simulink model "zoom_adc_single_pol"  (Simulink 7.8)
settings: Solver=FixedStepDiscrete  SolverMode=SingleTasking  StartTime=0.0  StopTime=4096  RelTol=1e-3
undefined symbols (not defined in the file): pfb_coeff_gen_calc
libraries: xbsIndex_r4 x1083, casper_library_misc x66, casper_library_delays x56, xps_library x25, simulink x1
(part 1 of 11)
settings Model: Creator=jayanth  LastModifiedBy=dprice
settings Model: ModifiedComment=|
  | dprice -- Tue Apr 16 12:08:08 2013 -- Version 1.114
  | 
  | First commit at Parkes, 16th April 2013. Just added in the FFT wideband black box, as I've tested this FFT and have faith that it works.
settings Model: ModifiedHistory=|
  | dprice -- Tue Apr 16 12:08:08 2013 -- Version 1.114
  | 
  | First commit at Parkes, 16th April 2013. Just added in the FFT wideband black box, as I've tested this FFT and have faith that it works.
settings DebuggingCC: FcnCallInpInsideContextMsg=Use local settings

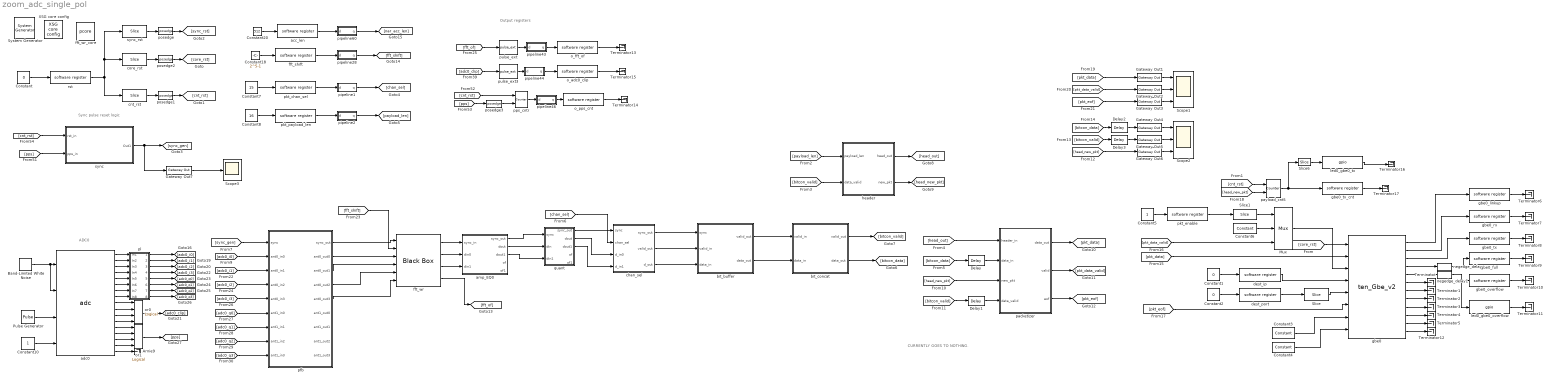
== system zoom_adc_single_pol ==
  note: Sync pulse reset logic
  note: CURRENTLY GOES TO NOTHING.
  note: ADC0
  note: Output registers
  " System Generator" : xbsIndex_r4/ System Generator  Tag=genX  xilinxfamily=virtex5  part=xc5vsx95t  speed=-1  package=ff1136  synthesis_tool=XST  clock_wrapper=Clock Enables  directory=./zoom_adc_single_pol/sysgen  proj_type=Project Navigator  Synth_file=XST Defaults  Impl_file=ISE Defaults  testbench=off  simulink_period=1  sysclk_period=5  dcm_input_clock_period=100  incr_netlist=off  trim_vbits=Everywhere in SubSystem  dbl_ovrd=According to Block Masks  core_generation=According to Block Masks  run_coregen=off  deprecated_control=off  eval_field=0  block_type=sysgen
  Arnie9 : Terminator
  Band-Limited White Noise : simulink/Sources/Band-Limited White Noise  Cov=[0.1]  Ts=0.1  seed=[23341]
  Constant : Constant  Value=0
  Constant1 : Constant  Value=0
  Constant10 : Constant
  Constant18 : Constant  Value=2^5-1
  Constant2 : Constant  Value=0
  Constant20 : Constant  Value=512
  Constant3 : xbsIndex_r4/Constant  const=1  gui_display_data_type=Boolean  arith_type=Boolean  n_bits=16  bin_pt=14  preci_type=Single  exp_width=8  frac_width=24  explicit_period=on  period=1  equ=P=C  opselect=C  inp2=PCIN>>17  opr=+  inp1=P  carry=CIN  dbl_ovrd=off  block_type=constant
  Constant4 : xbsIndex_r4/Constant  const=0  gui_display_data_type=Boolean  arith_type=Boolean  n_bits=16  bin_pt=14  preci_type=Single  exp_width=8  frac_width=24  explicit_period=on  period=1  equ=P=C  opselect=C  inp2=PCIN>>17  opr=+  inp1=P  carry=CIN  dbl_ovrd=off  block_type=constant
  Constant5 : Constant
  Constant6 : xbsIndex_r4/Constant  const=0  gui_display_data_type=Boolean  arith_type=Boolean  n_bits=16  bin_pt=14  preci_type=Single  exp_width=8  frac_width=24  explicit_period=off  period=1  equ=P=C  opselect=C  inp2=PCIN>>17  opr=+  inp1=P  carry=CIN  dbl_ovrd=off  block_type=constant
  Constant7 : Constant  Value=15
  Constant8 : Constant  Value=16
  Delay{,1..3} (4 alike) : xbsIndex_r4/Delay  rst=off  infoeditControl=Selection of Reset will increase slice count due to use of real FFs and instead of SRLs  en=off  latency=1  dbl_ovrd=off  reg_retiming=off  block_type=delay
  Gateway Out{1..7} (7 alike) : xbsIndex_r4/Gateway Out  inherit_from_input=off  hdl_port=on  timing_constraint=None  locs_specified=off  LOCs={}  UseAsDAC=off  DACChannel='1'  block_type=gatewayout
      settings: infoedit="Gateway out block.  Converts Xilinx fixed-point or floating-point type inputs into ouputs of type Simulink integer, single, double, or fixed point.<br><br>Hardware notes:  In hardware these blocks become top level output ports or are discarded, depending on how they are configured."
  Mux : xbsIndex_r4/Mux  inputs=2  en=off  latency=0  precision=Full  arith_type=Unsigned  n_bits=16  bin_pt=14  quantization=Truncate  overflow=Wrap  dbl_ovrd=off  block_type=mux
  Pulse Generator : DiscretePulseGenerator  PulseType=Time based  Period=10  PulseWidth=5
  Scope1 : Scope  NumInputPorts=3
      settings: TimeRange=290.1459854014598  YMin=9.44473e+21~0~-1  YMax=3.5e+38~1~1
  Scope2 : Scope  NumInputPorts=3
      settings: TimeRange=290.1459854014598  YMin=0~0~0  YMax=1.2e+18~1~1
  Scope3 : Scope
      settings: SaveName=ScopeData6
  Slice : xbsIndex_r4/Slice  nbits=16  boolean_output=off  mode=Lower Bit Location + Width  bit1=0  base1=MSB of Input  bit0=0  base0=LSB of Input  dbl_ovrd=off  block_type=slice
  Slice1 : xbsIndex_r4/Slice  nbits=1  boolean_output=on  mode=Lower Bit Location + Width  bit1=1  base1=MSB of Input  bit0=0  base0=LSB of Input  dbl_ovrd=off  block_type=slice
      settings: block_version=10.1.3
  Slice6 : xbsIndex_r4/Slice  nbits=1  boolean_output=on  mode=Lower Bit Location + Width  bit1=0  base1=MSB of Input  bit0=15  base0=LSB of Input  dbl_ovrd=off  block_type=slice
      settings: block_version=10.1.3
  Terminator{,1..17} (18 alike) : Terminator
  XSG core config : xps_library/XSG core config  Tag=xps:xsg  hw_sys=ROACH:sx95t  ibob_linux=off  clk_src=adc0_clk  iBOB_clk_src=sys_clk  BEE2_ctrl_clk_src=sys_clk  BEE2_usr_clk_src=sys_clk  ROACH_clk_src=adc0_clk  ROACH2_clk_src=adc0_clk  CORR_clk_src=sys_clk  gpio_clk_io_group=iBOB:sma  gpio_clk_bit_index=0  clk_rate=200  sample_period=1  synthesis_tool=XST  mpc_type=powerpc440_ext
  acc_len : xps_library/software register  Tag=xps:sw_reg  io_dir=From Processor  arith_type=Unsigned  bitwidth=32  bin_pt=0  sample_period=1  gw_name=zoom_adc_single_pol_acc_len_user_data_out
      link override coarse_r01_acc_len_user_data_out: arith_type=Unsigned  n_bits=32  bin_pt=0  period=1
      link override coarse_r02_acc_len_user_data_out: arith_type=Unsigned  n_bits=32  bin_pt=0  period=1
      link override coarse_r03_acc_len_user_data_out: arith_type=Unsigned  n_bits=32  bin_pt=0  period=1
      link override coarse_r04_acc_len_user_data_out: arith_type=Unsigned  n_bits=32  bin_pt=0  period=1
      link override coarse_r06_acc_len_user_data_out: arith_type=Unsigned  n_bits=32  bin_pt=0  period=1
      link override coarse_r07_acc_len_user_data_out: arith_type=Unsigned  n_bits=32  bin_pt=0  period=1
      link override coarse_r08_acc_len_user_data_out: arith_type=Unsigned  n_bits=32  bin_pt=0  period=1
      link override coarse_r09_acc_len_user_data_out: arith_type=Unsigned  n_bits=32  bin_pt=0  period=1
      link override coarse_r10_acc_len_user_data_out: arith_type=Unsigned  n_bits=32  bin_pt=0  period=1
      link override coarse_r12_acc_len_user_data_out: arith_type=Unsigned  n_bits=32  bin_pt=0  period=1
      link override convert: arith_type=Unsigned  n_bits=32  bin_pt=0
      link override qdr_single_r01_acc_len_coarse_user_data_out: arith_type=Unsigned  n_bits=32  bin_pt=0  period=1
      link override qdr_single_r02_acc_len_coarse_user_data_out: arith_type=Unsigned  n_bits=32  bin_pt=0  period=1
      link override qdr_single_r04_acc_len_coarse_user_data_out: arith_type=Unsigned  n_bits=32  bin_pt=0  period=1
      link override r_spec_2048_r102_acc_len_user_data_out: arith_type=Unsigned  n_bits=32  bin_pt=0  period=1
      link override r_spec_2048_r102_nosim_acc_len_user_data_out: arith_type=Unsigned  n_bits=32  bin_pt=0  period=1
      link override r_spec_2048_r103_acc_len_user_data_out: arith_type=Unsigned  n_bits=32  bin_pt=0  period=1
      link override r_spec_2048_r104_acc_len_user_data_out: arith_type=Unsigned  n_bits=32  bin_pt=0  period=1
      link override r_spec_2048_r104_test0_acc_len_user_data_out: arith_type=Unsigned  n_bits=32  bin_pt=0  period=1
      link override r_spec_2048_r104_test_acc_len_user_data_out: arith_type=Unsigned  n_bits=32  bin_pt=0  period=1
      link override r_spec_2048_r105_acc_len_user_data_out: arith_type=Unsigned  n_bits=32  bin_pt=0  period=1
      link override r_spec_test0_acc_len_user_data_out: arith_type=Unsigned  n_bits=32  bin_pt=0  period=1
      link override r_spec_test4_acc_len_user_data_out: arith_type=Unsigned  n_bits=32  bin_pt=0  period=1
      link override roach_spec_acc_len_user_data_out: arith_type=Unsigned  n_bits=32  bin_pt=0  period=1
      link override roach_spec_no10gbe_acc_len_user_data_out: arith_type=Unsigned  n_bits=32  bin_pt=0  period=1
      link override roach_spec_rst_sync_cnt_user_data_out: arith_type=Unsigned  n_bits=32  bin_pt=0  period=1
      link override toast_256ch_16bit_r02_acc_len_user_data_out: arith_type=Unsigned  n_bits=32  bin_pt=0  period=1
      link override toast_256ch_16bit_r04_acc_len_user_data_out: arith_type=Unsigned  n_bits=32  bin_pt=0  period=1
      link override toast_256ch_16bit_r05_acc_len_user_data_out: arith_type=Unsigned  n_bits=32  bin_pt=0  period=1
  adc0 : xps_library/adc  Tag=xps:adc  adc_brd=adc0  adc_clk_rate=800  adc_interleave=off  sample_period=1
  amp_EQ0 : Subsystem  mask{N=4, bram_lat=2, mult_lat=3, add_lat=2}
      mask prompts: N "number of coefficients (2^?)"; bram_lat "bram latency"; mult_lat "multiplier latency"; add_lat "adder latency"
  bit_buffer : Subsystem
  bit_concat : Subsystem
  chan_sel : Subsystem
  cnt_rst : xbsIndex_r4/Slice  nbits=1  boolean_output=on  mode=Lower Bit Location + Width  bit1=0  base1=MSB of Input  bit0=0  base0=LSB of Input  dbl_ovrd=off  block_type=slice
  core_rst : xbsIndex_r4/Slice  nbits=1  boolean_output=on  mode=Lower Bit Location + Width  bit1=0  base1=MSB of Input  bit0=1  base0=LSB of Input  dbl_ovrd=off  block_type=slice
  dest_ip : xps_library/software register  Tag=xps:sw_reg  io_dir=From Processor  arith_type=Unsigned  bitwidth=32  bin_pt=0  sample_period=1  gw_name=zoom_adc_single_pol_dest_ip_user_data_out
      link override hipsr_tgbe3_dest_ip_user_data_out: arith_type=Unsigned  n_bits=32  bin_pt=0  period=1
  dest_port : xps_library/software register  Tag=xps:sw_reg  io_dir=From Processor  arith_type=Unsigned  bitwidth=32  bin_pt=0  sample_period=1  gw_name=zoom_adc_single_pol_dest_port_user_data_out
      link override hipsr_tgbe3_dest_port_user_data_out: arith_type=Unsigned  n_bits=32  bin_pt=0  period=1
  fft_shift : xps_library/software register  Tag=xps:sw_reg  io_dir=From Processor  arith_type=Unsigned  bitwidth=32  bin_pt=0  sample_period=1  gw_name=zoom_adc_single_pol_fft_shift_user_data_out
      link override coarse_r01_acc_len_user_data_out: arith_type=Unsigned  n_bits=32  bin_pt=0  period=1
      link override coarse_r02_acc_len_user_data_out: arith_type=Unsigned  n_bits=32  bin_pt=0  period=1
      link override coarse_r03_acc_len_user_data_out: arith_type=Unsigned  n_bits=32  bin_pt=0  period=1
      link override coarse_r04_acc_len_user_data_out: arith_type=Unsigned  n_bits=32  bin_pt=0  period=1
      link override coarse_r06_acc_len_user_data_out: arith_type=Unsigned  n_bits=32  bin_pt=0  period=1
      link override coarse_r07_acc_len_user_data_out: arith_type=Unsigned  n_bits=32  bin_pt=0  period=1
      link override coarse_r08_acc_len_user_data_out: arith_type=Unsigned  n_bits=32  bin_pt=0  period=1
      link override coarse_r09_acc_len_user_data_out: arith_type=Unsigned  n_bits=32  bin_pt=0  period=1
      link override coarse_r10_acc_len_user_data_out: arith_type=Unsigned  n_bits=32  bin_pt=0  period=1
      link override coarse_r12_acc_len_user_data_out: arith_type=Unsigned  n_bits=32  bin_pt=0  period=1
      link override convert: arith_type=Unsigned  n_bits=32  bin_pt=0
      link override qdr_single_r01_acc_len_coarse_user_data_out: arith_type=Unsigned  n_bits=32  bin_pt=0  period=1
      link override qdr_single_r02_acc_len_coarse_user_data_out: arith_type=Unsigned  n_bits=32  bin_pt=0  period=1
      link override qdr_single_r04_acc_len_coarse_user_data_out: arith_type=Unsigned  n_bits=32  bin_pt=0  period=1
      link override r_spec_2048_r102_acc_len_user_data_out: arith_type=Unsigned  n_bits=32  bin_pt=0  period=1
      link override r_spec_2048_r102_nosim_acc_len_user_data_out: arith_type=Unsigned  n_bits=32  bin_pt=0  period=1
      link override r_spec_2048_r103_acc_len_user_data_out: arith_type=Unsigned  n_bits=32  bin_pt=0  period=1
      link override r_spec_2048_r104_acc_len_user_data_out: arith_type=Unsigned  n_bits=32  bin_pt=0  period=1
      link override r_spec_2048_r104_test0_acc_len_user_data_out: arith_type=Unsigned  n_bits=32  bin_pt=0  period=1
      link override r_spec_2048_r104_test_acc_len_user_data_out: arith_type=Unsigned  n_bits=32  bin_pt=0  period=1
      link override r_spec_2048_r105_acc_len_user_data_out: arith_type=Unsigned  n_bits=32  bin_pt=0  period=1
      link override r_spec_test0_acc_len_user_data_out: arith_type=Unsigned  n_bits=32  bin_pt=0  period=1
      link override r_spec_test4_acc_len_user_data_out: arith_type=Unsigned  n_bits=32  bin_pt=0  period=1
      link override roach_spec_acc_len_user_data_out: arith_type=Unsigned  n_bits=32  bin_pt=0  period=1
      link override roach_spec_no10gbe_acc_len_user_data_out: arith_type=Unsigned  n_bits=32  bin_pt=0  period=1
      link override roach_spec_rst_sync_cnt_user_data_out: arith_type=Unsigned  n_bits=32  bin_pt=0  period=1
      link override toast_256ch_16bit_r02_acc_len_user_data_out: arith_type=Unsigned  n_bits=32  bin_pt=0  period=1
      link override toast_256ch_16bit_r04_acc_len_user_data_out: arith_type=Unsigned  n_bits=32  bin_pt=0  period=1
      link override toast_256ch_16bit_r05_acc_len_user_data_out: arith_type=Unsigned  n_bits=32  bin_pt=0  period=1
  fft_wr : xbsIndex_r4/Black Box  init_code=fft_32pt_11x_core_config  sim_method=Inactive  verbose=off  block_type=blackbox2
  fft_wr_core : xps_library/pcore  Tag=xps:pcore  pcore_path=./bb/fft_32pt_11x_core/fft_32pt_11x_core.ngc
  gbe0 : xps_library/ten_Gbe_v2  Tag=xps:tengbe_v2  port=0  rx_dist_ram=off  large_frames=on  show_param=off  pre_emph=3  swing=800  fab_en=on  fab_mac=hex2dec('123456780000')  fab_ip=192*(2^24) + 168*(2^16) + 5*(2^8) + 20*(2^0)  fab_udp=10000  fab_gate=1  cpu_rx_en=on  cpu_tx_en=on
  gbe0_full : xps_library/software register  Tag=xps:sw_reg  io_dir=To Processor  arith_type=Unsigned  bitwidth=32  bin_pt=0  sample_period=1  gw_name=zoom_adc_single_pol_gbe0_full_user_data_in
      link override convert: arith_type=Unsigned  n_bits=32  bin_pt=0
  gbe0_linkup : xps_library/software register  Tag=xps:sw_reg  io_dir=To Processor  arith_type=Unsigned  bitwidth=32  bin_pt=0  sample_period=1  gw_name=zoom_adc_single_pol_gbe0_linkup_user_data_in
      link override convert: arith_type=Unsigned  n_bits=32  bin_pt=0
  gbe0_overflow : xps_library/software register  Tag=xps:sw_reg  io_dir=To Processor  arith_type=Unsigned  bitwidth=32  bin_pt=0  sample_period=1  gw_name=zoom_adc_single_pol_gbe0_overflow_user_data_in
      link override convert: arith_type=Unsigned  n_bits=32  bin_pt=0
  gbe0_rx : xps_library/software register  Tag=xps:sw_reg  io_dir=To Processor  arith_type=Unsigned  bitwidth=32  bin_pt=0  sample_period=1  gw_name=zoom_adc_single_pol_gbe0_rx_user_data_in
      link override convert: arith_type=Unsigned  n_bits=32  bin_pt=0
  gbe0_tx : xps_library/software register  Tag=xps:sw_reg  io_dir=To Processor  arith_type=Unsigned  bitwidth=32  bin_pt=0  sample_period=1  gw_name=zoom_adc_single_pol_gbe0_tx_user_data_in
      link override convert: arith_type=Unsigned  n_bits=32  bin_pt=0
  gbe0_tx_cnt : xps_library/software register  Tag=xps:sw_reg  io_dir=To Processor  arith_type=Unsigned  bitwidth=32  bin_pt=0  sample_period=1  gw_name=zoom_adc_single_pol_gbe0_tx_cnt_user_data_in
      link override convert: arith_type=Unsigned  n_bits=32  bin_pt=0
  header : Subsystem
  led0_gbe0_overflow : xps_library/gpio  Tag=xps:gpio  io_group=ROACH:led  io_dir=out  arith_type=Boolean  bitwidth=1  bin_pt=0  bit_index=1  sample_period=1  use_single_ended=off  use_ddr=off  reg_iob=on  reg_clk_phase=0  termination=None
      link override convert: arith_type=Boolean  n_bits=1  bin_pt=0
  led0_gbe0_tx : xps_library/gpio  Tag=xps:gpio  io_group=ROACH:led  io_dir=out  arith_type=Boolean  bitwidth=1  bin_pt=0  bit_index=0  sample_period=1  use_single_ended=off  use_ddr=off  reg_iob=off  reg_clk_phase=0  termination=None
      link override convert: arith_type=Boolean  n_bits=1  bin_pt=0
  negedge_delay : casper_library_misc/negedge_delay  pulse_len=2^20
  negedge_delay1 : casper_library_misc/negedge_delay  pulse_len=2^20
  o_adc0_clip : xps_library/software register  Tag=xps:sw_reg  io_dir=To Processor  arith_type=Unsigned  bitwidth=32  bin_pt=0  sample_period=1  gw_name=zoom_adc_single_pol_o_adc0_clip_user_data_in
      link override convert: arith_type=Unsigned  n_bits=32  bin_pt=0
  o_fft_of : xps_library/software register  Tag=xps:sw_reg  io_dir=To Processor  arith_type=Unsigned  bitwidth=32  bin_pt=0  sample_period=1  gw_name=zoom_adc_single_pol_o_fft_of_user_data_in
      link override convert: arith_type=Unsigned  n_bits=32  bin_pt=0
  o_pps_cnt : xps_library/software register  Tag=xps:sw_reg  io_dir=To Processor  arith_type=Unsigned  bitwidth=32  bin_pt=0  sample_period=1  gw_name=zoom_adc_single_pol_o_pps_cnt_user_data_in
      link override convert: arith_type=Unsigned  n_bits=32  bin_pt=0
  or0 : xbsIndex_r4/Logical  logical_function=OR  inputs=4  en=off  latency=2  precision=Full  arith_type=Unsigned  n_bits=16  bin_pt=0  align_bp=off  dbl_ovrd=off  block_type=logical
  or1 : xbsIndex_r4/Logical  logical_function=OR  inputs=4  en=off  latency=2  precision=Full  arith_type=Unsigned  n_bits=16  bin_pt=0  align_bp=off  dbl_ovrd=off  block_type=logical
  packetizer : Subsystem
  payload_cnt5 : xbsIndex_r4/Counter  cnt_type=Free Running  cnt_to=0  operation=Up  start_count=0  cnt_by_val=1  arith_type=Unsigned  n_bits=32  bin_pt=0  load_pin=off  rst=on  en=on  explicit_period=on  period=1  dbl_ovrd=off  use_behavioral_HDL=off  implementation=Fabric  use_rpm=on  block_type=counter
      settings: xl_area=[0, 0, 0, 0, 0, 0, 0]
  pfb : Subsystem
  pipeline1 : Subsystem  AncestorBlock=casper_library_delays/pipeline  mask(pipeline){latency=1}
      mask help:
      | An explicitly laid-out delay line to avoid mapping to SRL16s
      | for use in pipelining to help achieve timing closure.
      mask init:
      | pipeline_init(gcb,'latency',latency);
      settings: AttributesFormatString=Latency = %<latency>
      mask Display:
      | port_label('input', 1, 'd');
      | port_label('output', 1, 'q');
      | disp(['Z^-', num2str(latency)]);
  pipeline2 : Subsystem  AncestorBlock=casper_library_delays/pipeline  mask(pipeline){latency=1}
      mask help:
      | An explicitly laid-out delay line to avoid mapping to SRL16s
      | for use in pipelining to help achieve timing closure.
      mask init:
      | pipeline_init(gcb,'latency',latency);
      settings: AttributesFormatString=Latency = %<latency>
      mask Display:
      | port_label('input', 1, 'd');
      | port_label('output', 1, 'q');
      | disp(['Z^-', num2str(latency)]);
  pipeline28 : Subsystem  AncestorBlock=casper_library_delays/pipeline  mask(pipeline){latency=1}
      mask help:
      | An explicitly laid-out delay line to avoid mapping to SRL16s
      | for use in pipelining to help achieve timing closure.
      mask init:
      | pipeline_init(gcb,'latency',latency);
      settings: AttributesFormatString=Latency = %<latency>
      mask Display:
      | port_label('input', 1, 'd');
      | port_label('output', 1, 'q');
      | disp(['Z^-', num2str(latency)]);
  pipeline43 : Subsystem  AncestorBlock=casper_library_delays/pipeline  mask(pipeline){latency=1}
      mask help:
      | An explicitly laid-out delay line to avoid mapping to SRL16s
      | for use in pipelining to help achieve timing closure.
      mask init:
      | pipeline_init(gcb,'latency',latency);
      settings: AttributesFormatString=Latency = %<latency>
      mask Display:
      | port_label('input', 1, 'd');
      | port_label('output', 1, 'q');
      | disp(['Z^-', num2str(latency)]);
  pipeline44 : Subsystem  AncestorBlock=casper_library_delays/pipeline  mask(pipeline){latency=1}
      mask help:
      | An explicitly laid-out delay line to avoid mapping to SRL16s
      | for use in pipelining to help achieve timing closure.
      mask init:
      | pipeline_init(gcb,'latency',latency);
      settings: AttributesFormatString=Latency = %<latency>
      mask Display:
      | port_label('input', 1, 'd');
      | port_label('output', 1, 'q');
      | disp(['Z^-', num2str(latency)]);
  pipeline46 : Subsystem  AncestorBlock=casper_library_delays/pipeline  mask(pipeline){latency=1}
      mask help:
      | An explicitly laid-out delay line to avoid mapping to SRL16s
      | for use in pipelining to help achieve timing closure.
      mask init:
      | pipeline_init(gcb,'latency',latency);
      settings: AttributesFormatString=Latency = %<latency>
      mask Display:
      | port_label('input', 1, 'd');
      | port_label('output', 1, 'q');
      | disp(['Z^-', num2str(latency)]);
  pipeline60 : Subsystem  AncestorBlock=casper_library_delays/pipeline  mask(pipeline){latency=1}
      mask help:
      | An explicitly laid-out delay line to avoid mapping to SRL16s
      | for use in pipelining to help achieve timing closure.
      mask init:
      | pipeline_init(gcb,'latency',latency);
      settings: AttributesFormatString=Latency = %<latency>
      mask Display:
      | port_label('input', 1, 'd');
      | port_label('output', 1, 'q');
      | disp(['Z^-', num2str(latency)]);
  pkt_chan_sel : xps_library/software register  Tag=xps:sw_reg  io_dir=From Processor  arith_type=Unsigned  bitwidth=32  bin_pt=0  sample_period=1  gw_name=zoom_adc_single_pol_pkt_chan_sel_user_data_out
      link override hipsr_tgbe3_pkt_chan_sel_user_data_out: arith_type=Unsigned  n_bits=32  bin_pt=0  period=1
  pkt_enable : xps_library/software register  Tag=xps:sw_reg  io_dir=From Processor  arith_type=Unsigned  bitwidth=32  bin_pt=0  sample_period=1  gw_name=zoom_adc_single_pol_pkt_enable_user_data_out
      link override hipsr_tgbe3_pkt_enable_user_data_out: arith_type=Unsigned  n_bits=32  bin_pt=0  period=1
  pkt_payload_len : xps_library/software register  Tag=xps:sw_reg  io_dir=From Processor  arith_type=Unsigned  bitwidth=32  bin_pt=0  sample_period=1  gw_name=zoom_adc_single_pol_pkt_payload_len_user_data_out
      link override hipsr_tgbe3_pkt_payload_len_user_data_out: arith_type=Unsigned  n_bits=32  bin_pt=0  period=1
  pl : Subsystem
  posedge{,1..3} (4 alike) : casper_library_misc/posedge  Tag=Rising Edge Detector
  pps_cntr : xbsIndex_r4/Counter  cnt_type=Free Running  cnt_to=Inf  operation=Up  start_count=0  cnt_by_val=1  arith_type=Unsigned  n_bits=16  bin_pt=0  load_pin=off  rst=on  en=on  explicit_period=on  period=1  dbl_ovrd=off  use_behavioral_HDL=off  implementation=Fabric  use_rpm=off  block_type=counter
  pulse_ext : casper_library_misc/pulse_ext  pulse_len=100000
  pulse_ext3 : casper_library_misc/pulse_ext  pulse_len=100000
  quant : Subsystem
  rst : xps_library/software register  Tag=xps:sw_reg  io_dir=From Processor  arith_type=Unsigned  bitwidth=32  bin_pt=0  sample_period=1  gw_name=zoom_adc_single_pol_rst_user_data_out
      link override hipsr_tgbe3_rst_user_data_out: arith_type=Unsigned  n_bits=32  bin_pt=0  period=1
  sync : Subsystem  AncestorBlock=hipsr_library/sync
  sync_rst : xbsIndex_r4/Slice  nbits=1  boolean_output=on  mode=Lower Bit Location + Width  bit1=0  base1=MSB of Input  bit0=2  base0=LSB of Input  dbl_ovrd=off  block_type=slice
  wires:
  Constant/1 -> rst/1
  rst/1 -> cnt_rst/1, core_rst/1, sync_rst/1
  core_rst/1 -> posedge2/1
  cnt_rst/1 -> posedge1/1
  [core_rst] -> gbe0/1
  Constant2/1 -> dest_port/1
  Constant1/1 -> dest_ip/1
  dest_ip/1 -> gbe0/4
  dest_port/1 -> Slice/1
  Slice/1 -> gbe0/5
  gbe0/6 -> Terminator/1
  gbe0/7 -> Terminator1/1
  gbe0/8 -> Terminator2/1
  gbe0/9 -> Terminator3/1
  gbe0/10 -> Terminator4/1
  gbe0/11 -> Terminator5/1
  Constant3/1 -> gbe0/7
  gbe0/1 -> gbe0_linkup/1
  gbe0/2 -> gbe0_rx/1
  gbe0/3 -> gbe0_tx/1
  gbe0/4 -> negedge_delay/1
  negedge_delay/1 -> gbe0_full/1
  gbe0/5 -> negedge_delay1/1
  negedge_delay1/1 -> gbe0_overflow/1, led0_gbe0_overflow/1
  payload_cnt5/1 -> Slice6/1, gbe0_tx_cnt/1
  Slice6/1 -> led0_gbe0_tx/1
  [cnt_rst] -> payload_cnt5/1
  led0_gbe0_tx/1 -> Terminator16/1
  gbe0_tx_cnt/1 -> Terminator17/1
  gbe0_linkup/1 -> Terminator6/1
  gbe0_rx/1 -> Terminator7/1
  gbe0_tx/1 -> Terminator8/1
  gbe0_full/1 -> Terminator9/1
  gbe0_overflow/1 -> Terminator10/1
  led0_gbe0_overflow/1 -> Terminator11/1
  Constant4/1 -> gbe0/8
  gbe0/12 -> Terminator12/1
  sync_rst/1 -> posedge/1
  posedge/1 -> [sync_rst]
  posedge1/1 -> [cnt_rst]
  posedge2/1 -> [core_rst]
  Constant7/1 -> pkt_chan_sel/1
  pkt_chan_sel/1 -> pipeline1/1(d)
  Gateway Out4/1 -> Scope2/1
  Gateway Out5/1 -> Scope2/2
  Gateway Out6/1 -> Scope2/3
  Constant5/1 -> pkt_enable/1
  pkt_enable/1 -> Slice1/1
  Slice1/1 -> Mux/1
  Constant6/1 -> Mux/2
  Mux/1 -> gbe0/3
  [pkt_data] -> gbe0/2
  Constant8/1 -> pkt_payload_len/1
  pkt_payload_len/1 -> pipeline2/1(d)
  bit_buffer/1(valid_out) -> bit_concat/1(valid_in)
  bit_buffer/2(data_out) -> bit_concat/2(data_in)
  bit_concat/2(data_out) -> [bitcon_data]
  bit_concat/1(valid_out) -> [bitcon_valid]
  [payload_len] -> header/1(payload_len)
  [bitcon_valid] -> header/2(data_valid)
  header/1(head_out) -> [head_out]
  [head_out] -> packetizer/1(header_in)
  [bitcon_data] -> Delay/1
  header/2(new_pkt) -> [head_new_pkt]
  [head_new_pkt] -> packetizer/3(new_pkt)
  [bitcon_valid] -> Delay1/1
  packetizer/1(data_out) -> [pkt_data]
  packetizer/2(valid) -> [pkt_data_valid]
  packetizer/3(eof) -> [pkt_eof]
  [bitcon_data] -> Delay2/1
  [bitcon_valid] -> Delay3/1
  [head_new_pkt] -> Gateway Out6/1
  [pkt_data_valid] -> Mux/3
  [pkt_eof] -> gbe0/6
  [head_new_pkt] -> payload_cnt5/2
  Gateway Out1/1 -> Scope1/1
  Gateway Out2/1 -> Scope1/2
  Gateway Out3/1 -> Scope1/3
  [pkt_data] -> Gateway Out1/1
  [pkt_data_valid] -> Gateway Out2/1
  [pkt_eof] -> Gateway Out3/1
  Delay/1 -> packetizer/2(data_in)
  Delay1/1 -> packetizer/4(data_valid)
  Delay2/1 -> Gateway Out4/1
  Delay3/1 -> Gateway Out5/1
  pfb/2(ant0_out0) -> fft_wr/3
  pfb/3(ant0_out1) -> fft_wr/4
  pfb/4(ant0_out2) -> fft_wr/5
  pfb/5(ant0_out3) -> fft_wr/6
  pfb/1(sync_out) -> fft_wr/1
  fft_wr/4 -> [fft_of]
  [fft_shift] -> fft_wr/2
  [pps] -> sync/2(pps_in)
  sync/1(Out1) -> [sync_gen], Gateway Out7/1
  [cnt_rst] -> sync/1(rst_in)
  Gateway Out7/1 -> Scope3/1
  Constant18/1 -> fft_shift/1
  fft_shift/1 -> pipeline28/1(d)
  pipeline28/1(q) -> [fft_shift]
  Constant20/1 -> acc_len/1
  acc_len/1 -> pipeline60/1(d)
  pipeline60/1(q) -> [nar_acc_len]
  [chan_sel] -> chan_sel/2(chan_sel)
  chan_sel/1(sync_out) -> bit_buffer/1(sync)
  chan_sel/2(valid_out) -> bit_buffer/2(valid_in)
  chan_sel/3(d_out) -> bit_buffer/3(data_in)
  [sync_gen] -> pfb/1(sync)
  Band-Limited White Noise/1 -> adc0/1, adc0/2
  Pulse Generator/1 -> adc0/3
  Constant10/1 -> adc0/4
  adc0/9 -> or0/1
  adc0/10 -> or0/2
  adc0/11 -> or0/3
  adc0/12 -> or0/4
  adc0/13 -> or1/1
  adc0/14 -> or1/2
  adc0/15 -> or1/3
  adc0/16 -> or1/4
  adc0/17 -> Arnie9/1
  or0/1 -> [adc0_clip]
  or1/1 -> [pps]
  adc0/1 -> pl/1(In1)
  adc0/2 -> pl/2(In2)
  adc0/3 -> pl/3(In3)
  adc0/4 -> pl/4(In4)
  adc0/5 -> pl/5(In5)
  adc0/6 -> pl/6(In6)
  adc0/7 -> pl/7(In7)
  adc0/8 -> pl/8(In8)
  pl/1(Out1) -> [adc0_i0]
  pl/2(Out2) -> [adc0_i1]
  pl/3(Out3) -> [adc0_i2]
  pl/4(Out4) -> [adc0_i3]
  pl/5(Out5) -> [adc0_q0]
  pl/6(Out6) -> [adc0_q1]
  pl/7(Out7) -> [adc0_q2]
  pl/8(Out8) -> [adc0_q3]
  [adc0_q3] -> pfb/9(ant1_in3)
  [adc0_q2] -> pfb/8(ant1_in2)
  [adc0_q1] -> pfb/7(ant1_in1)
  [adc0_q0] -> pfb/6(ant1_in0)
  [adc0_i3] -> pfb/5(ant0_in3)
  [adc0_i2] -> pfb/4(ant0_in2)
  [adc0_i1] -> pfb/3(ant0_in1)
  [adc0_i0] -> pfb/2(ant0_in0)
  pipeline43/1(q) -> o_fft_of/1
  o_fft_of/1 -> Terminator13/1
  pipeline44/1(q) -> o_adc0_clip/1
  [adc0_clip] -> pulse_ext3/1
  o_adc0_clip/1 -> Terminator15/1
  pulse_ext3/1 -> pipeline44/1(d)
  [fft_of] -> pulse_ext/1
  pulse_ext/1 -> pipeline43/1(d)
  pps_cntr/1 -> pipeline46/1(d)
  pipeline46/1(q) -> o_pps_cnt/1
  o_pps_cnt/1 -> Terminator14/1
  [cnt_rst] -> pps_cntr/1
  posedge3/1 -> pps_cntr/2
  [pps] -> posedge3/1
  pipeline1/1(q) -> [chan_sel]
  pipeline2/1(q) -> [payload_len]
  fft_wr/1 -> amp_EQ0/1(sync_in)
  fft_wr/2 -> amp_EQ0/2(din0)
  fft_wr/3 -> amp_EQ0/3(din1)
  amp_EQ0/2(dout) -> quant/2(din)
  amp_EQ0/3(dout1) -> quant/3(din1)
  quant/2(dout) -> chan_sel/3(d_in0)
  quant/3(dout1) -> chan_sel/4(d_in1)
  amp_EQ0/1(sync_out) -> quant/1(sync)
  quant/1(sync_out) -> chan_sel/1(sync)

== system zoom_adc_single_pol/amp_EQ0 ==
  sync_in : Inport
  din0 : Inport  Port=2
  din1 : Inport  Port=3
  Constant : xbsIndex_r4/Constant  const=0  gui_display_data_type=Fixed-point  arith_type=Boolean  n_bits=16  bin_pt=14  preci_type=Single  exp_width=8  frac_width=24  explicit_period=on  period=1  equ=P=C  opselect=C  inp2=PCIN>>17  opr=+  inp1=P  carry=CIN  dbl_ovrd=off  block_type=constant
      settings: block_version=11.4
  Constant1 : xbsIndex_r4/Constant  const=0  gui_display_data_type=Fixed-point  arith_type=Unsigned  n_bits=32  bin_pt=0  preci_type=Single  exp_width=8  frac_width=24  explicit_period=on  period=1  equ=P=C  opselect=C  inp2=PCIN>>17  opr=+  inp1=P  carry=CIN  dbl_ovrd=off  block_type=constant
      settings: block_version=11.4
  Constant2 : xbsIndex_r4/Constant  const=0  gui_display_data_type=Fixed-point  arith_type=Boolean  n_bits=16  bin_pt=14  preci_type=Single  exp_width=8  frac_width=24  explicit_period=on  period=1  equ=P=C  opselect=C  inp2=PCIN>>17  opr=+  inp1=P  carry=CIN  dbl_ovrd=off  block_type=constant
      settings: block_version=11.4
  Constant3 : xbsIndex_r4/Constant  const=0  gui_display_data_type=Fixed-point  arith_type=Unsigned  n_bits=32  bin_pt=0  preci_type=Single  exp_width=8  frac_width=24  explicit_period=on  period=1  equ=P=C  opselect=C  inp2=PCIN>>17  opr=+  inp1=P  carry=CIN  dbl_ovrd=off  block_type=constant
      settings: block_version=11.4
  Counter : xbsIndex_r4/Counter  cnt_type=Free Running  cnt_to=Inf  operation=Up  start_count=0  cnt_by_val=1  arith_type=Unsigned  n_bits=N+1  bin_pt=0  load_pin=off  rst=on  en=off  explicit_period=on  period=1  dbl_ovrd=off  use_behavioral_HDL=off  implementation=Fabric  block_type=counter
      settings: block_version=11.4
  Delay : xbsIndex_r4/Delay  rst=off  infoeditControl=Selection of Reset will increase slice count due to use of real FFs and instead of SRLs  en=off  latency=6  dbl_ovrd=off  reg_retiming=off  block_type=delay
      settings: block_version=11.4
  Delay1 : xbsIndex_r4/Delay  rst=off  infoeditControl=Selection of Reset will increase slice count due to use of real FFs and instead of SRLs  en=off  latency=1  dbl_ovrd=off  reg_retiming=off  block_type=delay
      settings: block_version=11.4
  Delay2 : xbsIndex_r4/Delay  rst=off  infoeditControl=Selection of Reset will increase slice count due to use of real FFs and instead of SRLs  en=off  latency=1  dbl_ovrd=off  reg_retiming=off  block_type=delay
      settings: block_version=11.4
  Delay3 : xbsIndex_r4/Delay  rst=off  infoeditControl=Selection of Reset will increase slice count due to use of real FFs and instead of SRLs  en=off  latency=1  dbl_ovrd=off  reg_retiming=off  block_type=delay
      settings: block_version=11.4
  Slice : xbsIndex_r4/Slice  nbits=N  boolean_output=off  mode=Lower Bit Location + Width  bit1=0  base1=MSB of Input  bit0=1  base0=LSB of Input  dbl_ovrd=off  block_type=slice
  amp_scale : Subsystem
  amp_scale1 : Subsystem
  coeff_bram : Subsystem  Tag=xps:bram  AncestorBlock=xps_library/Shared BRAM  mask{arith_type=Unsigned, addr_width=max(N,10), data_width=32, data_bin_pt=0, init_vals=ones(2^N,1)*2, sample_rate=1}
      mask prompts: arith_type "Output Data Type"; addr_width "Address width"; data_width "Data Width"; data_bin_pt "Data Binary Point"; init_vals "Initial 32-bit values (simulation only)"; sample_rate "Sample rate"
      mask init:
      | shared_bram_mask;
      mask StyleString: popup(Unsigned|Signed  (2's comp)),edit,popup(8|16|32|64|128),edit,edit,edit
  coeff_bram1 : Subsystem  Tag=xps:bram  AncestorBlock=xps_library/Shared BRAM  mask{arith_type=Unsigned, addr_width=max(N,10), data_width=32, data_bin_pt=0, init_vals=ones(2^N,1)*2, sample_rate=1}
      mask prompts: arith_type "Output Data Type"; addr_width "Address width"; data_width "Data Width"; data_bin_pt "Data Binary Point"; init_vals "Initial 32-bit values (simulation only)"; sample_rate "Sample rate"
      mask init:
      | shared_bram_mask;
      mask StyleString: popup(Unsigned|Signed  (2's comp)),edit,popup(8|16|32|64|128),edit,edit,edit
  sync_out : Outport
  dout : Outport  Port=2
  dout1 : Outport  Port=3
  of : Outport  Port=4
  of1 : Outport  Port=5
  wires:
  coeff_bram/1(data_out) -> amp_scale/2(scale)
  Counter/1 -> Slice/1
  sync_in/1 -> Counter/1, Delay2/1
  din0/1 -> Delay1/1
  amp_scale/1(Out) -> dout/1
  Delay/1 -> sync_out/1
  amp_scale/2(of) -> of/1
  Delay1/1 -> amp_scale/1(din)
  Delay2/1 -> Delay/1
  Slice/1 -> coeff_bram/1(addr), coeff_bram1/1(addr)
  coeff_bram1/1(data_out) -> amp_scale1/2(scale)
  din1/1 -> Delay3/1
  amp_scale1/1(Out) -> dout1/1
  amp_scale1/2(of) -> of1/1
  Delay3/1 -> amp_scale1/1(din)
  Constant2/1 -> coeff_bram1/3(we)
  Constant3/1 -> coeff_bram1/2(data_in)
  Constant/1 -> coeff_bram/3(we)
  Constant1/1 -> coeff_bram/2(data_in)

== system zoom_adc_single_pol/bit_buffer ==
  sync : Inport
  valid_in : Inport  Port=2
  data_in : Inport  Port=3
  FIFO : xbsIndex_r4/FIFO  performance_options=Standard_FIFO  depth=16  percent_nbits=1  rst=on  en=off  use_dcount=off  use_percent_full_port=off  use_almost_empty=off  almost_empty_thresh=2  use_almost_full=off  almost_full_thresh=14  dbl_ovrd=off  mem_type=Block RAM  explicit_period=off  block_type=fifo
  Gateway Out{,1..3} (4 alike) : xbsIndex_r4/Gateway Out  inherit_from_input=off  hdl_port=on  timing_constraint=None  locs_specified=off  LOCs={}  UseAsDAC=off  DACChannel='1'  block_type=gatewayout
      settings: infoedit="Gateway out block.  Converts Xilinx fixed-point or floating-point type inputs into ouputs of type Simulink integer, single, double, or fixed point.<br><br>Hardware notes:  In hardware these blocks become top level output ports or are discarded, depending on how they are configured."
  Scope1 : Scope  NumInputPorts=2
      settings: YMin=-5~-5  YMax=5~5  SaveName=ScopeData3
  Scope2 : Scope  NumInputPorts=2
      settings: YMin=-5~-5  YMax=5~5  SaveName=ScopeData2
  fifo_re : Subsystem  mask{buf_len=2}
      mask prompts: buf_len "Buffer length (2^N)"
      mask help:
      | Read enabler block for FIFO buffer. Counts for desired number of valid datum,
      | then spits out data in a chunk.
  valid_out : Outport
  data_out : Outport  Port=2
  wires:
  data_in/1 -> FIFO/1, Gateway Out2/1
  valid_in/1 -> fifo_re/2(valid_in), FIFO/2, Gateway Out3/1
  sync/1 -> FIFO/4, fifo_re/1(rst)
  FIFO/1 -> data_out/1, Gateway Out/1
  fifo_re/1(re_out) -> FIFO/3, valid_out/1, Gateway Out1/1
  Gateway Out/1 -> Scope1/1
  Gateway Out1/1 -> Scope1/2
  Gateway Out2/1 -> Scope2/1
  Gateway Out3/1 -> Scope2/2

== system zoom_adc_single_pol/bit_concat ==
  valid_in : Inport
  data_in : Inport  Port=2
  Delay : xbsIndex_r4/Delay  rst=off  infoeditControl=Selection of Reset will increase slice count due to use of real FFs and instead of SRLs  en=off  latency=7  dbl_ovrd=off  reg_retiming=off  block_type=delay
  Gateway Out{,1..3} (4 alike) : xbsIndex_r4/Gateway Out  inherit_from_input=off  hdl_port=on  timing_constraint=None  locs_specified=off  LOCs={}  UseAsDAC=off  DACChannel='1'  block_type=gatewayout
      settings: infoedit="Gateway out block.  Converts Xilinx fixed-point or floating-point type inputs into ouputs of type Simulink integer, single, double, or fixed point.<br><br>Hardware notes:  In hardware these blocks become top level output ports or are discarded, depending on how they are configured."
  Scope : Scope  NumInputPorts=4
      settings: YMin=-5~-5~-5~-5  YMax=5~5~5~5  SaveName=ScopeData7
  cram : Subsystem  AncestorBlock=gavrt_library/cram  mask(cram){num_slice=4}
      mask prompts: num_slice "Number of slices"
      mask help: Concatenates inputs together after forcing binary point to zero.
      mask init:
      | cram_init(gcb, ...
      |     'num_slice', num_slice);
  delay_line : Subsystem
  posedge : casper_library_misc/posedge  Tag=Rising Edge Detector
  valid_out : Outport
  data_out : Outport  Port=2
  wires:
  data_in/1 -> delay_line/1(In1)
  delay_line/1(o1) -> cram/1(In1), Gateway Out1/1
  delay_line/2(o2) -> cram/2(In2), Gateway Out2/1
  delay_line/3(o3) -> cram/3(In3), Gateway Out3/1
  delay_line/4(o4) -> cram/4(In4)
  valid_in/1 -> posedge/1
  posedge/1 -> Delay/1
  Delay/1 -> valid_out/1, Gateway Out/1
  cram/1(Out) -> data_out/1
  Gateway Out/1 -> Scope/1
  Gateway Out1/1 -> Scope/2
  Gateway Out2/1 -> Scope/3
  Gateway Out3/1 -> Scope/4

== system zoom_adc_single_pol/chan_sel ==
  note: t
  sync : Inport
  chan_sel : Inport  Port=2
  d_in0 : Inport  Port=3
  d_in1 : Inport  Port=4
  Constant1 : xbsIndex_r4/Constant  const=0  gui_display_data_type=Fixed-point  arith_type=Boolean  n_bits=1  bin_pt=0  preci_type=Single  exp_width=8  frac_width=24  explicit_period=on  period=1  equ=P=C  opselect=C  inp2=PCIN>>17  opr=+  inp1=P  carry=CIN  dbl_ovrd=off  block_type=constant
  Constant2 : xbsIndex_r4/Constant  const=1  gui_display_data_type=Boolean  arith_type=Boolean  n_bits=1  bin_pt=0  preci_type=Single  exp_width=8  frac_width=24  explicit_period=on  period=1  equ=P=C  opselect=C  inp2=PCIN>>17  opr=+  inp1=P  carry=CIN  dbl_ovrd=off  block_type=constant
  Delay1 : xbsIndex_r4/Delay  rst=off  infoeditControl=Selection of Reset will increase slice count due to use of real FFs and instead of SRLs  en=off  latency=1  dbl_ovrd=off  reg_retiming=on  block_type=delay
      settings: xl_area=[0, 0, 0, 0, 0, 0, 0]
  Delay5 : xbsIndex_r4/Delay  rst=off  infoeditControl=Selection of Reset will increase slice count due to use of real FFs and instead of SRLs  en=off  latency=1  dbl_ovrd=off  reg_retiming=on  block_type=delay
      settings: xl_area=[0, 0, 0, 0, 0, 0, 0]
  Mux : xbsIndex_r4/Mux  inputs=2  en=off  latency=1  precision=Full  arith_type="Signed  (2's comp)"  n_bits=8  bin_pt=2  quantization=Truncate  overflow=Wrap  dbl_ovrd=off  block_type=mux
      settings: xl_area=[0, 0, 0, 0, 0, 0, 0]
  Mux1 : xbsIndex_r4/Mux  inputs=2  en=off  latency=0  precision=Full  arith_type=Unsigned  n_bits=16  bin_pt=14  quantization=Truncate  overflow=Wrap  dbl_ovrd=off  block_type=mux
  Slice : xbsIndex_r4/Slice  nbits=1  boolean_output=off  mode=Lower Bit Location + Width  bit1=0  base1=MSB of Input  bit0=0  base0=LSB of Input  dbl_ovrd=off  block_type=slice
  Slice2 : xbsIndex_r4/Slice  nbits=4  boolean_output=off  mode=Lower Bit Location + Width  bit1=1  base1=MSB of Input  bit0=1  base0=LSB of Input  dbl_ovrd=off  block_type=slice
      settings: block_version=10.1.3
  chan_cnt : xbsIndex_r4/Counter  cnt_type=Free Running  cnt_to=Inf  operation=Up  start_count=0  cnt_by_val=1  arith_type=Unsigned  n_bits=4  bin_pt=0  load_pin=off  rst=on  en=off  explicit_period=on  period=1  dbl_ovrd=off  use_behavioral_HDL=off  implementation=Fabric  block_type=counter
  chan_rel : xbsIndex_r4/Relational  mode=a=b  en=off  latency=0  dbl_ovrd=off  block_type=relational
  sync_out : Outport
  valid_out : Outport  Port=2
  d_out : Outport  Port=3
  wires:
  Delay5/1 -> d_out/1  "d_out"
  Mux/1 -> valid_out/1  "valid"
  Constant1/1 -> Mux/2
  sync/1 -> chan_cnt/1, Delay1/1
  chan_cnt/1 -> chan_rel/1
  Slice2/1 -> chan_rel/2
  Constant2/1 -> Mux/3
  chan_rel/1 -> Mux/1
  chan_sel/1 -> Slice2/1, Slice/1
  Delay1/1 -> sync_out/1
  d_in0/1 -> Mux1/2
  d_in1/1 -> Mux1/3
  Mux1/1 -> Delay5/1
  Slice/1 -> Mux1/1

== system zoom_adc_single_pol/header ==
  payload_len : Inport
  data_valid : Inport  Port=2
  Counter : xbsIndex_r4/Counter  cnt_type=Free Running  cnt_to=Inf  operation=Up  start_count=0  cnt_by_val=1  arith_type=Unsigned  n_bits=16  bin_pt=0  load_pin=off  rst=on  en=on  explicit_period=on  period=1  dbl_ovrd=off  use_behavioral_HDL=off  implementation=Fabric  block_type=counter
  Counter2 : xbsIndex_r4/Counter  cnt_type=Free Running  cnt_to=Inf  operation=Up  start_count=0  cnt_by_val=1  arith_type=Unsigned  n_bits=32  bin_pt=0  load_pin=off  rst=off  en=on  explicit_period=on  period=1  dbl_ovrd=off  use_behavioral_HDL=off  implementation=Fabric  block_type=counter
  Relational : xbsIndex_r4/Relational  mode=a=b  en=off  latency=0  dbl_ovrd=off  block_type=relational
  head_struct : Subsystem
  head_out : Outport
  new_pkt : Outport  Port=2
  wires:
  Counter/1 -> Relational/2
  Relational/1 -> Counter/1, Counter2/1, new_pkt/1
  Counter2/1 -> head_struct/1(pkt_num)
  head_struct/1(data_out) -> head_out/1
  payload_len/1 -> Relational/1
  data_valid/1 -> Counter/2

== system zoom_adc_single_pol/packetizer ==
  header_in : Inport
  data_in : Inport  Port=2
  new_pkt : Inport  Port=3
  data_valid : Inport  Port=4
  Constant : xbsIndex_r4/Constant  const=1  gui_display_data_type=Boolean  arith_type=Boolean  n_bits=16  bin_pt=14  preci_type=Single  exp_width=8  frac_width=24  explicit_period=on  period=1  equ=P=C  opselect=C  inp2=PCIN>>17  opr=+  inp1=P  carry=CIN  dbl_ovrd=off  block_type=constant
  Delay1 : xbsIndex_r4/Delay  rst=off  infoeditControl=Selection of Reset will increase slice count due to use of real FFs and instead of SRLs  en=off  latency=4  dbl_ovrd=off  reg_retiming=off  block_type=delay
  Delay2 : xbsIndex_r4/Delay  rst=off  infoeditControl=Selection of Reset will increase slice count due to use of real FFs and instead of SRLs  en=off  latency=4  dbl_ovrd=off  reg_retiming=off  block_type=delay
  Mux : xbsIndex_r4/Mux  inputs=2  en=off  latency=0  precision=Full  arith_type=Unsigned  n_bits=16  bin_pt=14  quantization=Truncate  overflow=Wrap  dbl_ovrd=off  block_type=mux
  Mux1 : xbsIndex_r4/Mux  inputs=2  en=off  latency=0  precision=Full  arith_type=Unsigned  n_bits=16  bin_pt=14  quantization=Truncate  overflow=Wrap  dbl_ovrd=off  block_type=mux
  data_out : Outport
  valid : Outport  Port=2
  eof : Outport  Port=3
  wires:
  new_pkt/1 -> eof/1, Delay1/1
  header_in/1 -> Delay2/1
  data_in/1 -> Mux/2
  data_valid/1 -> Mux1/2
  Constant/1 -> Mux1/3
  Mux1/1 -> valid/1
  Mux/1 -> data_out/1
  Delay2/1 -> Mux/3
  Delay1/1 -> Mux/1, Mux1/1

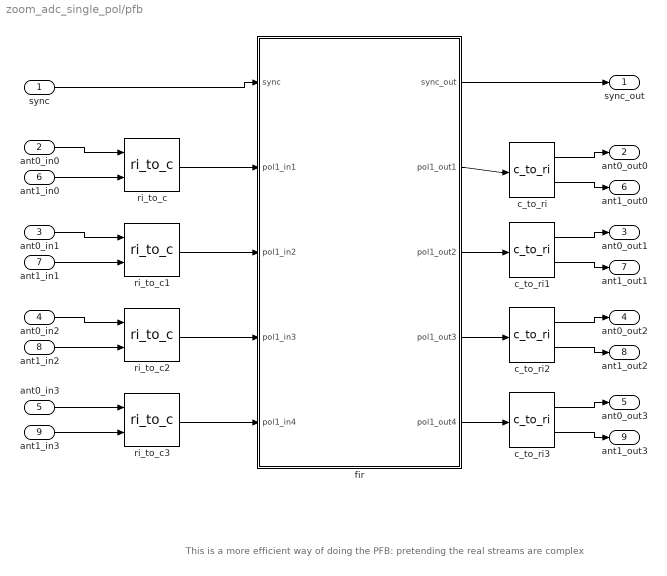
== system zoom_adc_single_pol/pfb ==
  note: This is a more efficient way of doing the PFB: pretending the real streams are complex
  sync : Inport
  ant0_in0 : Inport  Port=2
  ant0_in1 : Inport  Port=3
  ant0_in2 : Inport  Port=4
  ant0_in3 : Inport  Port=5
  ant1_in0 : Inport  Port=6
  ant1_in1 : Inport  Port=7
  ant1_in2 : Inport  Port=8
  ant1_in3 : Inport  Port=9
  c_to_ri{,1..3} (4 alike) : casper_library_misc/c_to_ri  n_bits=18  bin_pt=17
  fir : Subsystem  AncestorBlock=casper_library_pfbs/pfb_fir  mask(pfb_fir){PFBSize=5, TotalTaps=8, WindowType=hamming, n_inputs=2, MakeBiplex=0, BitWidthIn=8, BitWidthOut=18, CoeffBitWidth=25, CoeffDistMem=1, add_latency=1, mult_latency=2, bram_latency=2, quantization=Round  (unbiased: +/- Inf), fwidth=1, specify_mult=off, mult_spec=[2                                      2]}
      mask prompts: PFBSize "Size of PFB: (2^? pnts)"; TotalTaps "Total Number of Taps:"; WindowType "Windowing Function:"; n_inputs "Number of Simultaneous Inputs: (2^?)"; MakeBiplex "Make Biplex"; BitWidthIn "Input Bitwidth:"; BitWidthOut "Output Bitwidth:"; CoeffBitWidth "Coefficient Bitwidth:"; CoeffDistMem "Use Distributed Memory for Coeffs"; add_latency "Add Latency"; mult_latency "Mult Latency"; bram_latency "BRAM Latency"; quantization "Quantization Behavior"; fwidth "Bin Width Scaling (normal=1)"; specify_mult "Specify multiplier use (behavioral if not specified)"; mult_spec "Multiplier specification (0=core, 1=embedded, 2=behavioural) (left=1st tap)"
      mask init:
      | pfb_fir_init(gcb, ...
      |     'PFBSize', PFBSize, ...
      |     'TotalTaps', TotalTaps, ...
      |     'WindowType', WindowType, ...
      |     'n_inputs', n_inputs, ...
      |     'MakeBiplex', MakeBiplex, ...
      |     'BitWidthIn', BitWidthIn, ...
      |     'BitWidthOut', BitWidthOut, ...
      |     'CoeffBitWidth', CoeffBitWidth, ...
      |     'CoeffDistMem', CoeffDistMem, ...
      |     'add_latency', add_latency, ...
      |     'mult_latency', mult_latency, ...
      |     'bram_latency', bram_latency, ...
      |     'quantization', quantization, ...
      |     'fwidth', fwidth,...
      |     'specify_mult', specify_mult,...
      |     'mult_spec', mult_spec);
      settings: AttributesFormatString=|
      | taps=8, add_latency=1
      | max scale 0.822
      mask Help: eval('xlWeb(''http://casper.berkeley.edu/wiki/Pfb_fir'')')
      mask StyleString: edit,edit,popup(bartlett|barthannwin|blackman|blackmanharris|bohamwin|chebwin|flattopwin|gausswin|hamming|hann|kaiser|nuttallwin|parzenwin|rectwin|tukeywin|triang|userwindow),edit,edit,edit,edit,edit,edit,edit,edit,edit,popup(Truncate|Round  (unbiased: +/- Inf)|Round  (unbiased: Even Values)),edit,checkbox,edit
      mask CallbackString:
      | |%num_taps = eval(get_param(gcb, 'TotalTaps'));
      | %old_vec = eval(get_param(gcb, 'mult_spec'));
      | 
      | %vec = 2.*ones(1,num_taps);
      | %old_size = length(old_vec);
      | 
      | %if(old_size <= num_taps),
      | %   new_size = old_size;
      | %else,
      | %    new_size = num_taps;
      | %end
      | 
      | %for n = 1:new_size, vec(n) = old_vec(n); end
      | %set_param(gcb, 'mult_spec', mat2str(vec));||||||||||||%num_taps = eval(get_param(gcb, 'TotalTaps'));
      | %old_vec = eval(get_param(gcb, 'mult_spec'));
      | 
      | %vec = 2.*ones(1,num_taps);
      | %old_size = length(old_vec);
      | 
      | %if(old_size <= num_taps),
      | %    new_size = old_size;
      | %else,
      | %    new_size = num_taps;
      | %end
      | 
      | %for n = 1:new_size, vec(n) = old_vec(n); end
      | %set_param(gcb, 'mult_spec', mat2str(vec));|%specify_mult = get_param(gcb,'specify_mult');
      | %if( strcmp(specify_mult,'off')),
      | %    set_param(gcb, 'MaskEnables', {'on','on','on','on','on','on','on','on','on','on','on','on','on','on','on','off'});
      | %else
      | %    set_param(gcb, 'MaskEnables', {'on','on','on','on','on','on','on','on','on','on','on','on','on','on','on','on'});
      | %end
      | 
      | |%specify_mult = get_param(gcb,'specify_mult');
      | %if( strcmp(specify_mult,'off')),
      | %    set_param(gcb, 'MaskEnables', {'on','on','on','on','on','on','on','on','on','on','on','on','on','on','on','off'});
      | %else
      | %    set_param(gcb, 'MaskEnables', {'on','on','on','on','on','on','on','on','on','on','on','on','on','on','on','on'});
      | %end
  ri_to_c{,1..3} (4 alike) : casper_library_misc/ri_to_c
  sync_out : Outport
  ant0_out0 : Outport  Port=2
  ant0_out1 : Outport  Port=3
  ant0_out2 : Outport  Port=4
  ant0_out3 : Outport  Port=5
  ant1_out0 : Outport  Port=6
  ant1_out1 : Outport  Port=7
  ant1_out2 : Outport  Port=8
  ant1_out3 : Outport  Port=9
  wires:
  sync/1 -> fir/1(sync)
  fir/2(pol1_out1) -> c_to_ri/1
  fir/1(sync_out) -> sync_out/1
  c_to_ri/1 -> ant0_out0/1
  c_to_ri/2 -> ant1_out0/1
  c_to_ri1/1 -> ant0_out1/1
  c_to_ri1/2 -> ant1_out1/1
  c_to_ri2/1 -> ant0_out2/1
  c_to_ri2/2 -> ant1_out2/1
  c_to_ri3/1 -> ant0_out3/1
  c_to_ri3/2 -> ant1_out3/1
  fir/3(pol1_out2) -> c_to_ri1/1
  fir/4(pol1_out3) -> c_to_ri2/1
  fir/5(pol1_out4) -> c_to_ri3/1
  ant0_in0/1 -> ri_to_c/1
  ant1_in0/1 -> ri_to_c/2
  ant0_in1/1 -> ri_to_c1/1
  ant1_in1/1 -> ri_to_c1/2
  ant0_in2/1 -> ri_to_c2/1
  ant1_in2/1 -> ri_to_c2/2
  ant0_in3/1 -> ri_to_c3/1
  ant1_in3/1 -> ri_to_c3/2
  ri_to_c/1 -> fir/2(pol1_in1)
  ri_to_c1/1 -> fir/3(pol1_in2)
  ri_to_c2/1 -> fir/4(pol1_in3)
  ri_to_c3/1 -> fir/5(pol1_in4)

== system zoom_adc_single_pol/pipeline1 ==
  d : Inport
  Register0 : xbsIndex_r4/Register  init=0  rst=off  en=off  dbl_ovrd=off  block_type=register
      settings: block_version=11.4
  q : Outport
  wires:
  d/1 -> Register0/1
  Register0/1 -> q/1

== system zoom_adc_single_pol/pipeline2 ==
  d : Inport
  Register0 : xbsIndex_r4/Register  init=0  rst=off  en=off  dbl_ovrd=off  block_type=register
      settings: block_version=11.4
  q : Outport
  wires:
  d/1 -> Register0/1
  Register0/1 -> q/1

== system zoom_adc_single_pol/pipeline28 ==
  d : Inport
  Register0 : xbsIndex_r4/Register  init=0  rst=off  en=off  dbl_ovrd=off  block_type=register
      settings: block_version=11.4
  q : Outport
  wires:
  d/1 -> Register0/1
  Register0/1 -> q/1

== system zoom_adc_single_pol/pipeline43 ==
  d : Inport
  Register0 : xbsIndex_r4/Register  init=0  rst=off  en=off  dbl_ovrd=off  block_type=register
      settings: block_version=11.4
  q : Outport
  wires:
  d/1 -> Register0/1
  Register0/1 -> q/1

== system zoom_adc_single_pol/pipeline44 ==
  d : Inport
  Register0 : xbsIndex_r4/Register  init=0  rst=off  en=off  dbl_ovrd=off  block_type=register
      settings: block_version=11.4
  q : Outport
  wires:
  d/1 -> Register0/1
  Register0/1 -> q/1

== system zoom_adc_single_pol/pipeline46 ==
  d : Inport
  Register0 : xbsIndex_r4/Register  init=0  rst=off  en=off  dbl_ovrd=off  block_type=register
      settings: block_version=11.4
  q : Outport
  wires:
  d/1 -> Register0/1
  Register0/1 -> q/1

== system zoom_adc_single_pol/pipeline60 ==
  d : Inport
  Register0 : xbsIndex_r4/Register  init=0  rst=off  en=off  dbl_ovrd=off  block_type=register
      settings: block_version=11.4
  q : Outport
  wires:
  d/1 -> Register0/1
  Register0/1 -> q/1
